simulink model "q03"  (R2024a)
settings: Solver=VariableStepDiscrete  StartTime=0.0  StopTime=10.0  MaxStep=0.1  RelTol=1e-3
settings Model: Creator=amir  LastModifiedBy=amir

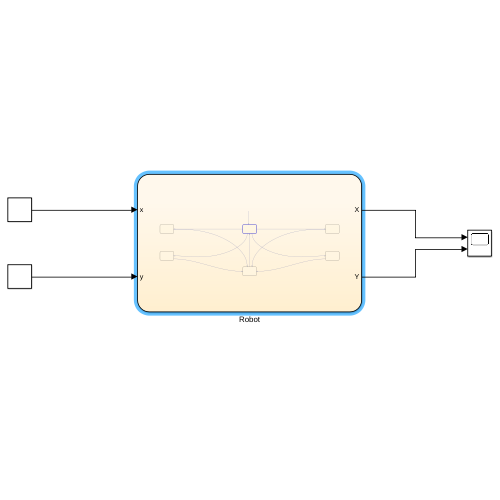
[thumbnail: Simulink's stored preview of the top-level diagram]
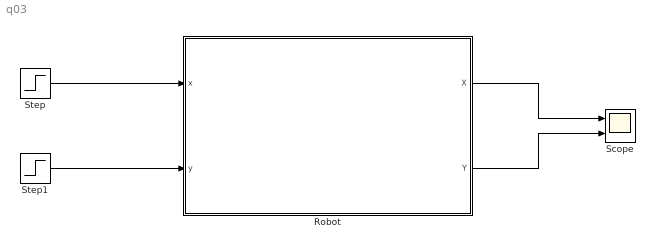
== system q03 ==
  Robot : Stateflow chart  TreatAsAtomicUnit=on
  Scope : Scope  NumInputPorts=2
  Step : Step  After=4  SampleTime=0
  Step1 : Step  After=10  SampleTime=0
  wires:
  Robot/1(X) -> Scope/1
  Robot/2(Y) -> Scope/2
  Step/1 -> Robot/1(x)
  Step1/1 -> Robot/2(y)

== stateflow chart q03/Robot ==
  state Down
  state Stopped
  state Up
  state Left
  state Right
  state Straight
  (default) -> Stopped : /{X = 0; Y = 0;}
  Stopped -> Down [order 2] : [(abs(Y-y) > 0.75 * abs(X-x)) && (y < Y)]/{Y = Y - (abs(Y-y) - 0.75 * abs(X-x))}
  Stopped -> Up [order 1] : [(abs(Y-y) > 0.75 * abs(X-x)) && (y > Y)]/{Y = Y + (abs(Y-y) - 0.75 * abs(X-x))}
  Down -> Straight : /{X = x; Y = y;}
  Up -> Straight : /{X = x; Y = y;}
  Stopped -> Left [order 3] : [(abs(Y-y) < 0.75 * abs(X-x)) && (x > X)]{X = X - (abs(X-x) - (4/3) * abs(Y-y))}
  Straight -> Stopped
  Stopped -> Right [order 4] : [(abs(Y-y) < 0.75 * abs(X-x)) && (x > X)]{X = X + (abs(X-x) - (4/3) * abs(Y-y))}
  Left -> Straight : /{X = x; Y = y;}
  Right -> Straight : /{X = x; Y = y;}
  data: x input; y input; X output; Y output
